simulink library "ddm"  (R2021b)
settings: Solver=VariableStepAuto  StartTime=0.0  StopTime=10.0  RelTol=1e-3
undefined symbols (not defined in the file or in its folder): ADDM_FrTMTqDev_X_Nm, ADDM_RrTMTqDev_X_Nm, ENUM_ADASACCSTA_ERROR, ENUM_ADASACCSTA_OFF, ENUM_ADASACCSTA_STANDBY, ENUM_ALLOWMOV_ALLOWREADY, ENUM_APS, ENUM_BRKSTA_ERROR, ENUM_BRKSTA_OFF, ENUM_BRKSTA_ON, ENUM_BRKSW_INVALID, ENUM_BRKSW_OFF, ENUM_BRKSW_ON, ENUM_CHGPREACTERRSTA_OBCPRE, ENUM_DCDCFAULTSTA_ANYFAULTLV1, ENUM_DCDCFAULTSTA_ANYFAULTLV2, ENUM_DRIVETRAIN_AWD, ENUM_DRIVETRAIN_FWD, ENUM_DRIVETRAIN_RWD, ENUM_EDUDRTSTA_NORMAL, ENUM_EPBSTA_APPLIED, ENUM_EPBSTA_RELEASED, ENUM_ESCAPSSta_APSUNAVAILABLE, ENUM_GEARACTUALPOSN_INVALID, ENUM_GEARACTUALPOSN_P, ENUM_HVBATTREADYPRE_READY, ENUM_MCUWARN_LV0, ENUM_MCUWARN_LV1, ENUM_MCUWARN_LV2, ENUM_MCUWARN_LV3, ENUM_MCUWARN_NOERROR, ENUM_OBCFAULTSTA_ANYFAULT, ENUM_PAS_R2F2, ENUM_PDFAULT_BATTPDFAIL, ENUM_PDFAULT_DCDCDISABLE, ENUM_PDFAULT_MCUDISABLE, ENUM_PDFAULT_MCUDISCHRG, ENUM_POWERSTA_OFF, ENUM_POWERSTA_ON, ENUM_POWERSTA_READY, ENUM_POWERSTA_STANDBY, ENUM_PRESSINDI_LOW, ENUM_PUFAULT_BATTUPFAIL, ENUM_PUFAULT_DCDCENABLEFAIL, ENUM_PUFAULT_PRECHRGCHKFAIL, ENUM_PUFAULT_SAFETYCHKFAIL, ENUM_PUSTATE_COMPLETED, ENUM_PWRSTASW_OFF, ENUM_PWRSTASW_OFFA, ENUM_PWRSTASW_OFFCHVCHRG, ENUM_PWRSTASW_OFFCLVCHRG, ENUM_PWRSTASW_ON, ENUM_PWRSTASW_ONHVCHRG, ENUM_PWRSTASW_READY, ENUM_PWRSTASW_STANDBY, ENUM_RAPSErrWarnSta_NORMAL, ENUM_RAPSErrWarnSta_RAPSERRLV1, ENUM_SHIFTCOMMAND_P, ENUM_SHIFTERERRSTA_PBUTTONFAILURE, ENUM_VEHMALFUNLV_2ND ... (+463)
libraries: hcu_lib x529, $bdroot x5, simulink x4
(part 18 of 25)

== system ddm/DDM/DDM/PMM/Comm err/VCU lost communication with ABM1 ==
  note: Test Detection Criteria
  note: Test Pass Criteria
  note: Release Condition After Decision
  note: Diagnostics and Fault Handling
  task_time_s : Inport
  VPMM_PowerSta_enum : Inport  Port=2
  VPMM_PwrStaSW_enum : Inport  Port=3
  VDDM_C1ABM1LCChk_flg : Inport  Port=4
  No_CAN1_BUS_OFF : Inport  Port=5
  DTC_clear_request : Inport  Port=6
  Constant1 : Constant  Value=ENUM_PWRSTASW_OFF
  Constant10 : Constant  Value=ENUM_POWERSTA_STANDBY
  Constant11 : Constant  Value=ZERO_INT
  Constant12 : Constant  Value=KDDM_C1ABM1LCDTC_cnt
  Constant13 : Constant  Value=FALSE
  Constant14 : Constant  Value=KDDM_C1ABM1LCDetTO_s
  Constant17 : Constant  Value=KDDM_C1ABM1LCDTC_cnt
  Constant29 : Constant  Value=FALSE
  Constant30 : Constant  Value=KDDM_CommErrDiagnosisOffSW_flg
  Constant31 : Constant  Value=ENUM_POWERSTA_OFF
  Constant6 : Constant  Value=KDDM_C1ABM1LCPassTO_s
  Constant7 : Constant  Value=TRUE
  Constant8 : Constant  Value=KDDM_C1ABM1LCPassTO_s
  Constant9 : Constant  Value=ENUM_PWRSTASW_OFF
  DTC_Couter1 : hcu_lib/Basic_Blocks/DTC_Couter
  DTC_Info : hcu_lib/Basic_Blocks/DTC_Info
  Equal1 : RelationalOperator  Operator=~=  OutDataTypeStr=boolean  RndMeth=Simplest
  Equal5 : RelationalOperator  Operator=~=  OutDataTypeStr=boolean  RndMeth=Simplest
  Equal6 : RelationalOperator  OutDataTypeStr=boolean  RndMeth=Simplest
  Equal7 : RelationalOperator  Operator===  OutDataTypeStr=boolean  RndMeth=Simplest
  Equal8 : RelationalOperator  Operator===  OutDataTypeStr=boolean  RndMeth=Simplest
  Logical Operator1 : Logic  Operator=NOT  AllPortsSameDT=off  OutDataTypeStr=boolean
  Logical Operator10 : Logic  AllPortsSameDT=off  OutDataTypeStr=boolean
  Logical Operator14 : Logic  Operator=OR  Inputs=4  AllPortsSameDT=off  OutDataTypeStr=boolean
  Logical Operator16 : Logic  AllPortsSameDT=off  OutDataTypeStr=boolean
  Logical Operator20 : Logic  Operator=NOT  AllPortsSameDT=off  OutDataTypeStr=boolean
  Logical Operator3 : Logic  Operator=NOT  AllPortsSameDT=off  OutDataTypeStr=boolean
  Logical Operator9 : Logic  AllPortsSameDT=off  OutDataTypeStr=boolean
  Relational Operator1 : RelationalOperator  Operator=>  OutDataTypeStr=boolean  RndMeth=Simplest
  Switch2 : Switch  Criteria=u2 ~= 0
  Switch8 : Switch  Criteria=u2 ~= 0
  Switch9 : Switch  Criteria=u2 ~= 0
  Terminator : Terminator
  Test Detection Criteria1 : hcu_lib/Basic_Blocks/Test Detection Criteria
  Timer2 : hcu_lib/Basic_Blocks/Timer
  Unit Delay1 : UnitDelay  SampleTime=-1  HasFrameUpgradeWarning=on
  VDDM_C1ABM1LCDTC_raw32 : Outport
  VDDM_C1ABM1LCCFS_flg : Outport  Port=2
  LC_EDriveSysErr_VCUErr_flg : Outport  Port=3
  wires:
  [DTC_clear_request] -> DTC_Info/4
  [VDDM_C1ABM1LCPass_flg] -> DTC_Info/2
  [VDDM_C1ABM1LCDet_flg] -> DTC_Info/1
  [VDDM_C1ABM1LCCFS_flg] -> DTC_Info/3
  DTC_Info/1 -> VDDM_C1ABM1LCDTC_raw32/1  "VDDM_C1ABM1LCDTC_raw32"
  [VDDM_C1ABM1LCCFS_flg] -> LC_EDriveSysErr_VCUErr_flg/1, VDDM_C1ABM1LCCFS_flg/1
  No_CAN1_BUS_OFF/1 -> [No_CAN1_BUS_OFF]
  DTC_clear_request/1 -> [DTC_clear_request]
  task_time_s/1 -> [task_time_s]
  VDDM_C1ABM1LCChk_flg/1 -> [VDDM_C1ABM1LCChk_flg]
  VPMM_PwrStaSW_enum/1 -> [VPMM_PwrStaSW_enum]
  VPMM_PowerSta_enum/1 -> [VPMM_PowerSta_enum]
  [VDDM_C1ABM1LCCFSRls_flg] -> Switch9/2
  [VDDM_C1ABM1LCChk_flg] -> Logical Operator1/1
  [VDDM_C1ABM1LCChk_flg] -> Logical Operator3/1
  [VDDM_C1ABM1LCCFSRls_flg] -> DTC_Couter1/2
  [task_time_s] -> Test Detection Criteria1/2
  Logical Operator20/1 -> Timer2/1
  [VPMM_PwrStaSW_enum] -> Equal5/1
  Logical Operator10/1 -> Switch8/2
  [No_CAN1_BUS_OFF] -> Logical Operator10/1
  Constant1/1 -> Equal5/2
  Relational Operator1/1 -> Terminator/1  "VDDM_C1ABM1LCDFS_flg"
  Constant6/1 -> Timer2/4
  Constant14/1 -> Test Detection Criteria1/4
  Constant10/1 -> Equal8/2
  Logical Operator16/1 -> Logical Operator14/1
  Equal7/1 -> Logical Operator16/1
  Constant12/1 -> Test Detection Criteria1/3
  [task_time_s] -> Timer2/3
  Equal5/1 -> Logical Operator10/2
  Equal6/1 -> [VDDM_C1ABM1LCPass_flg]  "VDDM_C1ABM1LCPass_flg"
  Constant17/1 -> DTC_Couter1/3
  Equal8/1 -> Logical Operator16/2
  Constant11/1 -> Relational Operator1/2
  [No_CAN1_BUS_OFF] -> Logical Operator9/1
  [VDDM_C1ABM1LCPass_flg] -> Logical Operator14/3
  Switch9/1 -> Test Detection Criteria1/1
  [VDDM_C1ABM1LCDet_flg] -> DTC_Couter1/1
  Constant31/1 -> Equal7/2
  DTC_Couter1/2 -> Relational Operator1/1  "VDDM_C1ABM1LCDTC_cnt"
  DTC_Couter1/1 -> [VDDM_C1ABM1LCCFS_flg]  "VDDM_C1ABM1LCCFS_flg"
  Unit Delay1/1 -> Equal7/1
  Constant13/1 -> Switch2/3
  [DTC_clear_request] -> Logical Operator14/2
  Constant9/1 -> Equal1/2
  Constant8/1 -> Equal6/2
  Constant7/1 -> Switch8/3
  [VPMM_PowerSta_enum] -> Equal8/1
  Timer2/1 -> Equal6/1
  [VPMM_PwrStaSW_enum] -> Equal1/1
  Logical Operator14/1 -> [VDDM_C1ABM1LCCFSRls_flg]  "VDDM_C1ABM1LCCFSRls_flg"
  Constant30/1 -> Logical Operator14/4
  Switch8/1 -> Timer2/2, Logical Operator20/1
  Logical Operator9/1 -> Switch2/2
  Test Detection Criteria1/1 -> [VDDM_C1ABM1LCDet_flg]  "VDDM_C1ABM1LCDet_flg"
  Constant29/1 -> Switch9/1
  Equal1/1 -> Logical Operator9/2
  [VPMM_PowerSta_enum] -> Unit Delay1/1
  Switch2/1 -> Switch9/3
  Logical Operator3/1 -> Switch2/1
  Logical Operator1/1 -> Switch8/1

== system ddm/DDM/DDM/PMM/Comm err/VCU lost communication with BMS1 ==
  note: Test Pass Criteria
  note: Test Detection Criteria
  note: Diagnostics and Fault Handling
  note: Release Condition After Decision
  task_time_s : Inport
  VPMM_PowerSta_enum : Inport  Port=2
  VPMM_PwrStaSW_enum : Inport  Port=3
  VDDM_C3BMS1LCChk_flg : Inport  Port=4
  No_CAN3_BUS_OFF : Inport  Port=5
  DTC_clear_request : Inport  Port=6
  Constant1 : Constant  Value=ENUM_PWRSTASW_OFF
  Constant10 : Constant  Value=ENUM_POWERSTA_STANDBY
  Constant11 : Constant  Value=ZERO_INT
  Constant12 : Constant  Value=KDDM_C3BMS1LCPassTO_s
  Constant13 : Constant  Value=FALSE
  Constant14 : Constant  Value=KDDM_C3BMS1LCDTC_cnt
  Constant17 : Constant  Value=KDDM_C3BMS1LCDetTO_s
  Constant29 : Constant  Value=FALSE
  Constant30 : Constant  Value=KDDM_CommErrDiagnosisOffSW_flg
  Constant31 : Constant  Value=ENUM_POWERSTA_OFF
  Constant6 : Constant  Value=KDDM_C3BMS1LCDTC_cnt
  Constant7 : Constant  Value=TRUE
  Constant8 : Constant  Value=KDDM_C3BMS1LCPassTO_s
  Constant9 : Constant  Value=ENUM_PWRSTASW_OFF
  DTC_Couter1 : hcu_lib/Basic_Blocks/DTC_Couter
  DTC_Info : hcu_lib/Basic_Blocks/DTC_Info
  Delay1 : Delay  DelayLength=1
  Equal1 : RelationalOperator  Operator=~=  OutDataTypeStr=boolean  RndMeth=Simplest
  Equal5 : RelationalOperator  Operator=~=  OutDataTypeStr=boolean  RndMeth=Simplest
  Equal6 : RelationalOperator  OutDataTypeStr=boolean  RndMeth=Simplest
  Equal7 : RelationalOperator  Operator===  OutDataTypeStr=boolean  RndMeth=Simplest
  Equal8 : RelationalOperator  Operator===  OutDataTypeStr=boolean  RndMeth=Simplest
  Logical Operator : Logic  Operator=NOT  AllPortsSameDT=off  OutDataTypeStr=boolean
  Logical Operator14 : Logic  Operator=OR  Inputs=4  AllPortsSameDT=off  OutDataTypeStr=boolean
  Logical Operator{7,9,16,22} (4 alike) : Logic  AllPortsSameDT=off  OutDataTypeStr=boolean
  Logical Operator2 : Logic  Operator=NOT  AllPortsSameDT=off  OutDataTypeStr=boolean
  Logical Operator20 : Logic  Operator=NOT  AllPortsSameDT=off  OutDataTypeStr=boolean
  NOT1 : Logic  Operator=NOT  AllPortsSameDT=off  OutDataTypeStr=boolean
  Relational Operator1 : RelationalOperator  Operator=>  OutDataTypeStr=boolean  RndMeth=Simplest
  Switch2 : Switch  Criteria=u2 ~= 0
  Switch8 : Switch  Criteria=u2 ~= 0
  Switch9 : Switch  Criteria=u2 ~= 0
  Terminator : Terminator
  Test Detection Criteria1 : hcu_lib/Basic_Blocks/Test Detection Criteria
  Timer2 : hcu_lib/Basic_Blocks/Timer
  Unit Delay1 : UnitDelay  SampleTime=-1  HasFrameUpgradeWarning=on
  VDDM_C3BMS1LCDTC_raw32 : Outport
  VDDM_C3BMS1LCCFS_flg : Outport  Port=2
  wires:
  [VDDM_C3BMS1LCCFS_flg] -> Delay1/1
  Logical Operator20/1 -> Timer2/1
  Logical Operator14/1 -> [VDDM_C3BMS1LCCFSRls_flg]  "VDDM_C3BMS1LCCFSRls_flg"
  [task_time_s] -> Test Detection Criteria1/2
  Timer2/1 -> Equal6/1
  Test Detection Criteria1/1 -> [VDDM_C3BMS1LCDet_flg]  "VDDM_C3BMS1LCDet_flg"
  Equal1/1 -> Logical Operator7/2
  Constant9/1 -> Equal1/2
  Constant10/1 -> Equal8/2
  Constant8/1 -> Timer2/4
  Relational Operator1/1 -> Terminator/1  "VDDM_C3BMS1LCDFS_flg"
  Constant1/1 -> Equal5/2
  [No_CAN3_BUS_OFF] -> Logical Operator7/1
  Logical Operator16/1 -> Logical Operator14/1
  [VPMM_PwrStaSW_enum] -> Equal1/1
  DTC_Couter1/1 -> [VDDM_C3BMS1LCCFS_flg]  "VDDM_C3BMS1LCCFS_flg"
  [VPMM_PwrStaSW_enum] -> Equal5/1
  Equal5/1 -> Logical Operator9/2
  [No_CAN3_BUS_OFF] -> Logical Operator9/1
  Logical Operator7/1 -> Switch2/2
  [VDDM_C3BMS1LCPass_flg] -> Logical Operator22/1
  Delay1/1 -> NOT1/1
  Constant12/1 -> Equal6/2
  Unit Delay1/1 -> Equal7/1
  [VDDM_C3BMS1LCChk_flg] -> Logical Operator2/1
  Switch2/1 -> Switch9/3
  [task_time_s] -> Timer2/3
  [VDDM_C3BMS1LCDet_flg] -> DTC_Couter1/1
  Logical Operator9/1 -> Switch8/2
  [VDDM_C3BMS1LCChk_flg] -> Logical Operator/1
  [VDDM_C3BMS1LCCFSRls_flg] -> Switch9/2
  Equal6/1 -> [VDDM_C3BMS1LCPass_flg]  "VDDM_C3BMS1LCPass_flg"
  Constant6/1 -> DTC_Couter1/3
  Constant7/1 -> Switch8/3
  Logical Operator22/1 -> Logical Operator14/3
  Switch9/1 -> Test Detection Criteria1/1
  Constant30/1 -> Logical Operator14/4
  Equal8/1 -> Logical Operator16/2
  Constant29/1 -> Switch9/1
  NOT1/1 -> Logical Operator22/2
  [VPMM_PowerSta_enum] -> Equal8/1
  Constant13/1 -> Switch2/3
  Constant11/1 -> Relational Operator1/2
  DTC_Couter1/2 -> Relational Operator1/1  "VDDM_C3BMS1LCDTC_cnt"
  [DTC_clear_request] -> Logical Operator14/2
  Switch8/1 -> Logical Operator20/1, Timer2/2
  Constant31/1 -> Equal7/2
  [VPMM_PowerSta_enum] -> Unit Delay1/1
  Equal7/1 -> Logical Operator16/1
  [VDDM_C3BMS1LCCFSRls_flg] -> DTC_Couter1/2
  Constant14/1 -> Test Detection Criteria1/3
  Constant17/1 -> Test Detection Criteria1/4
  [VDDM_C3BMS1LCCFS_flg] -> DTC_Info/3, VDDM_C3BMS1LCCFS_flg/1
  task_time_s/1 -> [task_time_s]
  VDDM_C3BMS1LCChk_flg/1 -> [VDDM_C3BMS1LCChk_flg]
  VPMM_PwrStaSW_enum/1 -> [VPMM_PwrStaSW_enum]
  VPMM_PowerSta_enum/1 -> [VPMM_PowerSta_enum]
  No_CAN3_BUS_OFF/1 -> [No_CAN3_BUS_OFF]
  DTC_clear_request/1 -> [DTC_clear_request]
  DTC_Info/1 -> VDDM_C3BMS1LCDTC_raw32/1  "VDDM_C3BMS1LCDTC_raw32"
  [VDDM_C3BMS1LCDet_flg] -> DTC_Info/1
  [VDDM_C3BMS1LCPass_flg] -> DTC_Info/2
  [DTC_clear_request] -> DTC_Info/4
  Logical Operator/1 -> Switch2/1
  Logical Operator2/1 -> Switch8/1

== system ddm/DDM/DDM/PMM/Comm err/VCU lost communication with BMS6 ==
  note: Test Detection Criteria
  note: Release Condition After Decision
  note: Diagnostics and Fault Handling
  note: Test Pass Criteria
  task_time_s : Inport
  VPMM_PowerSta_enum : Inport  Port=2
  VPMM_PwrStaSW_enum : Inport  Port=3
  VDDM_C3BMS6LCChk_flg : Inport  Port=4
  No_CAN3_BUS_OFF : Inport  Port=5
  DTC_clear_request : Inport  Port=6
  Constant1 : Constant  Value=ENUM_PWRSTASW_OFF
  Constant10 : Constant  Value=ENUM_POWERSTA_STANDBY
  Constant11 : Constant  Value=ZERO_INT
  Constant12 : Constant  Value=KDDM_C3BMS6LCPassTO_s
  Constant13 : Constant  Value=FALSE
  Constant14 : Constant  Value=KDDM_C3BMS6LCDTC_cnt
  Constant17 : Constant  Value=KDDM_C3BMS6LCDetTO_s
  Constant27 : Constant  Value=KDDM_C3BMS6LCDTC_cnt
  Constant30 : Constant  Value=KDDM_CommErrDiagnosisOffSW_flg
  Constant31 : Constant  Value=ENUM_POWERSTA_OFF
  Constant6 : Constant  Value=TRUE
  Constant7 : Constant  Value=KDDM_C3BMS6LCPassTO_s
  Constant8 : Constant  Value=ENUM_PWRSTASW_OFF
  Constant9 : Constant  Value=FALSE
  DTC_Couter1 : hcu_lib/Basic_Blocks/DTC_Couter
  DTC_Info : hcu_lib/Basic_Blocks/DTC_Info
  Delay1 : Delay  DelayLength=1
  Equal1 : RelationalOperator  Operator=~=  OutDataTypeStr=boolean  RndMeth=Simplest
  Equal5 : RelationalOperator  Operator=~=  OutDataTypeStr=boolean  RndMeth=Simplest
  Equal6 : RelationalOperator  OutDataTypeStr=boolean  RndMeth=Simplest
  Equal7 : RelationalOperator  Operator===  OutDataTypeStr=boolean  RndMeth=Simplest
  Equal8 : RelationalOperator  Operator===  OutDataTypeStr=boolean  RndMeth=Simplest
  Logical Operator : Logic  Operator=NOT  AllPortsSameDT=off  OutDataTypeStr=boolean
  Logical Operator14 : Logic  Operator=OR  Inputs=4  AllPortsSameDT=off  OutDataTypeStr=boolean
  Logical Operator{7,9,16,22} (4 alike) : Logic  AllPortsSameDT=off  OutDataTypeStr=boolean
  Logical Operator2 : Logic  Operator=NOT  AllPortsSameDT=off  OutDataTypeStr=boolean
  Logical Operator20 : Logic  Operator=NOT  AllPortsSameDT=off  OutDataTypeStr=boolean
  NOT1 : Logic  Operator=NOT  AllPortsSameDT=off  OutDataTypeStr=boolean
  Relational Operator1 : RelationalOperator  Operator=>  OutDataTypeStr=boolean  RndMeth=Simplest
  Switch2 : Switch  Criteria=u2 ~= 0
  Switch8 : Switch  Criteria=u2 ~= 0
  Switch9 : Switch  Criteria=u2 ~= 0
  Terminator : Terminator
  Test Detection Criteria1 : hcu_lib/Basic_Blocks/Test Detection Criteria
  Timer2 : hcu_lib/Basic_Blocks/Timer
  Unit Delay1 : UnitDelay  SampleTime=-1  HasFrameUpgradeWarning=on
  VDDM_C3BMS6LCDTC_raw32 : Outport
  VDDM_C3BMS6LCCFS_flg : Outport  Port=2
  wires:
  Equal5/1 -> Logical Operator9/2
  Constant1/1 -> Equal5/2
  [No_CAN3_BUS_OFF] -> Logical Operator9/1
  [VPMM_PwrStaSW_enum] -> Equal5/1
  Equal1/1 -> Logical Operator7/2
  [VPMM_PwrStaSW_enum] -> Equal1/1
  Constant8/1 -> Equal1/2
  [No_CAN3_BUS_OFF] -> Logical Operator7/1
  [task_time_s] -> Timer2/3
  Timer2/1 -> Equal6/1
  [VDDM_C3BMS6LCChk_flg] -> Logical Operator/1
  Logical Operator20/1 -> Timer2/1
  Logical Operator16/1 -> Logical Operator14/1
  Relational Operator1/1 -> Terminator/1  "VDDM_C3BMS6LCDFS_flg"
  Constant27/1 -> DTC_Couter1/3
  Test Detection Criteria1/1 -> [VDDM_C3BMS6LCDet_flg]  "VDDM_C3BMS6LCDet_flg"
  [VDDM_C3BMS6LCChk_flg] -> Logical Operator2/1
  [VDDM_C3BMS6LCCFS_flg] -> Delay1/1
  Equal7/1 -> Logical Operator16/1
  Equal6/1 -> [VDDM_C3BMS6LCPass_flg]  "VDDM_C3BMS6LCPass_flg"
  [VPMM_PowerSta_enum] -> Unit Delay1/1
  [VDDM_C3BMS6LCDet_flg] -> DTC_Couter1/1
  DTC_Couter1/1 -> [VDDM_C3BMS6LCCFS_flg]  "VDDM_C3BMS6LCCFS_flg"
  Constant31/1 -> Equal7/2
  [VDDM_C3BMS6LCPass_flg] -> Logical Operator22/1
  Constant17/1 -> Test Detection Criteria1/4
  Constant14/1 -> Test Detection Criteria1/3
  Unit Delay1/1 -> Equal7/1
  Switch8/1 -> Logical Operator20/1, Timer2/2
  [DTC_clear_request] -> Logical Operator14/2
  Constant7/1 -> Timer2/4
  [VDDM_C3BMS6LCCFSRls_flg] -> DTC_Couter1/2
  Delay1/1 -> NOT1/1
  DTC_Couter1/2 -> Relational Operator1/1  "VDDM_C3BMS6LCDTC_cnt"
  Constant11/1 -> Relational Operator1/2
  Constant13/1 -> Switch2/3
  Logical Operator9/1 -> Switch8/2
  Constant10/1 -> Equal8/2
  Constant9/1 -> Switch9/1
  Switch2/1 -> Switch9/3
  [task_time_s] -> Test Detection Criteria1/2
  [VPMM_PowerSta_enum] -> Equal8/1
  Equal8/1 -> Logical Operator16/2
  Logical Operator7/1 -> Switch2/2
  NOT1/1 -> Logical Operator22/2
  Logical Operator22/1 -> Logical Operator14/3
  Constant6/1 -> Switch8/3
  Constant30/1 -> Logical Operator14/4
  Switch9/1 -> Test Detection Criteria1/1
  Logical Operator14/1 -> [VDDM_C3BMS6LCCFSRls_flg]  "VDDM_C3BMS6LCCFSRls_flg"
  Constant12/1 -> Equal6/2
  [VDDM_C3BMS6LCCFSRls_flg] -> Switch9/2
  VPMM_PowerSta_enum/1 -> [VPMM_PowerSta_enum]
  VPMM_PwrStaSW_enum/1 -> [VPMM_PwrStaSW_enum]
  VDDM_C3BMS6LCChk_flg/1 -> [VDDM_C3BMS6LCChk_flg]
  task_time_s/1 -> [task_time_s]
  [VDDM_C3BMS6LCCFS_flg] -> DTC_Info/3, VDDM_C3BMS6LCCFS_flg/1
  DTC_clear_request/1 -> [DTC_clear_request]
  No_CAN3_BUS_OFF/1 -> [No_CAN3_BUS_OFF]
  [VDDM_C3BMS6LCPass_flg] -> DTC_Info/2
  DTC_Info/1 -> VDDM_C3BMS6LCDTC_raw32/1  "VDDM_C3BMS6LCDTC_raw32"
  [VDDM_C3BMS6LCDet_flg] -> DTC_Info/1
  [DTC_clear_request] -> DTC_Info/4
  Logical Operator/1 -> Switch2/1
  Logical Operator2/1 -> Switch8/1

== system ddm/DDM/DDM/PMM/Comm err/VCU lost communication with CCU1 ==
  note: Diagnostics and Fault Handling
  note: Test Pass Criteria
  note: Test Detection Criteria
  note: Release Condition After Decision
  task_time_s : Inport
  VPMM_PowerSta_enum : Inport  Port=2
  VPMM_PwrStaSW_enum : Inport  Port=3
  VDDM_C3CCU1LCChk_flg : Inport  Port=4
  No_CAN3_BUS_OFF : Inport  Port=5
  DTC_clear_request : Inport  Port=6
  Constant1 : Constant  Value=ENUM_PWRSTASW_OFF
  Constant10 : Constant  Value=ENUM_POWERSTA_STANDBY
  Constant11 : Constant  Value=ZERO_INT
  Constant12 : Constant  Value=KDDM_C3CCU1LCPassTO_s
  Constant13 : Constant  Value=FALSE
  Constant14 : Constant  Value=KDDM_C3CCU1LCDTC_cnt
  Constant17 : Constant  Value=KDDM_C3CCU1LCDetTO_s
  Constant29 : Constant  Value=FALSE
  Constant30 : Constant  Value=KDDM_CommErrDiagnosisOffSW_flg
  Constant31 : Constant  Value=ENUM_POWERSTA_OFF
  Constant32 : Constant  Value=KDDM_C3CCU1LCDTC_cnt
  Constant7 : Constant  Value=TRUE
  Constant8 : Constant  Value=KDDM_C3CCU1LCPassTO_s
  Constant9 : Constant  Value=ENUM_PWRSTASW_OFF
  DTC_Couter1 : hcu_lib/Basic_Blocks/DTC_Couter
  DTC_Info : hcu_lib/Basic_Blocks/DTC_Info
  Delay1 : Delay  DelayLength=1
  Equal1 : RelationalOperator  Operator=~=  OutDataTypeStr=boolean  RndMeth=Simplest
  Equal5 : RelationalOperator  Operator=~=  OutDataTypeStr=boolean  RndMeth=Simplest
  Equal6 : RelationalOperator  OutDataTypeStr=boolean  RndMeth=Simplest
  Equal7 : RelationalOperator  Operator===  OutDataTypeStr=boolean  RndMeth=Simplest
  Equal8 : RelationalOperator  Operator===  OutDataTypeStr=boolean  RndMeth=Simplest
  Logical Operator1 : Logic  Operator=NOT  AllPortsSameDT=off  OutDataTypeStr=boolean
  Logical Operator14 : Logic  Operator=OR  Inputs=4  AllPortsSameDT=off  OutDataTypeStr=boolean
  Logical Operator{7,9,16,22} (4 alike) : Logic  AllPortsSameDT=off  OutDataTypeStr=boolean
  Logical Operator2 : Logic  Operator=NOT  AllPortsSameDT=off  OutDataTypeStr=boolean
  Logical Operator20 : Logic  Operator=NOT  AllPortsSameDT=off  OutDataTypeStr=boolean
  NOT1 : Logic  Operator=NOT  AllPortsSameDT=off  OutDataTypeStr=boolean
  Relational Operator1 : RelationalOperator  Operator=>  OutDataTypeStr=boolean  RndMeth=Simplest
  Switch2 : Switch  Criteria=u2 ~= 0
  Switch8 : Switch  Criteria=u2 ~= 0
  Switch9 : Switch  Criteria=u2 ~= 0
  Terminator : Terminator
  Test Detection Criteria1 : hcu_lib/Basic_Blocks/Test Detection Criteria
  Timer2 : hcu_lib/Basic_Blocks/Timer
  Unit Delay1 : UnitDelay  SampleTime=-1  HasFrameUpgradeWarning=on
  VDDM_C3CCU1LCDTC_raw32 : Outport
  VDDM_C3CCU1LCCFS_flg : Outport  Port=2
  wires:
  [DTC_clear_request] -> DTC_Info/4
  [VDDM_C3CCU1LCDet_flg] -> DTC_Info/1
  [VDDM_C3CCU1LCCFS_flg] -> VDDM_C3CCU1LCCFS_flg/1, DTC_Info/3
  [VDDM_C3CCU1LCPass_flg] -> DTC_Info/2
  DTC_Info/1 -> VDDM_C3CCU1LCDTC_raw32/1  "VDDM_C3CCU1LCDTC_raw32"
  No_CAN3_BUS_OFF/1 -> [No_CAN3_BUS_OFF]
  DTC_clear_request/1 -> [DTC_clear_request]
  task_time_s/1 -> [task_time_s]
  VDDM_C3CCU1LCChk_flg/1 -> [VDDM_C3CCU1LCChk_flg]
  VPMM_PwrStaSW_enum/1 -> [VPMM_PwrStaSW_enum]
  VPMM_PowerSta_enum/1 -> [VPMM_PowerSta_enum]
  Constant8/1 -> Timer2/4
  Relational Operator1/1 -> Terminator/1  "VDDM_C3CCU1LCDFS_flg"
  [No_CAN3_BUS_OFF] -> Logical Operator9/1
  Test Detection Criteria1/1 -> [VDDM_C3CCU1LCDet_flg]  "VDDM_C3CCU1LCDet_flg"
  Logical Operator16/1 -> Logical Operator14/1
  Constant10/1 -> Equal8/2
  [VPMM_PwrStaSW_enum] -> Equal1/1
  [task_time_s] -> Timer2/3
  Constant12/1 -> Equal6/2
  Switch2/1 -> Switch9/3
  Equal5/1 -> Logical Operator9/2
  Logical Operator7/1 -> Switch2/2
  Delay1/1 -> NOT1/1
  Constant32/1 -> DTC_Couter1/3
  Constant7/1 -> Switch8/3
  Constant30/1 -> Logical Operator14/4
  Constant29/1 -> Switch9/1
  [VPMM_PowerSta_enum] -> Equal8/1
  Constant13/1 -> Switch2/3
  Switch9/1 -> Test Detection Criteria1/1
  DTC_Couter1/1 -> [VDDM_C3CCU1LCCFS_flg]  "VDDM_C3CCU1LCCFS_flg"
  Logical Operator22/1 -> Logical Operator14/3
  Equal8/1 -> Logical Operator16/2
  Constant11/1 -> Relational Operator1/2
  NOT1/1 -> Logical Operator22/2
  [DTC_clear_request] -> Logical Operator14/2
  Unit Delay1/1 -> Equal7/1
  DTC_Couter1/2 -> Relational Operator1/1  "VDDM_C3CCU1LCDTC_cnt"
  Timer2/1 -> Equal6/1
  Constant31/1 -> Equal7/2
  [VPMM_PowerSta_enum] -> Unit Delay1/1
  Switch8/1 -> Timer2/2, Logical Operator20/1
  Constant17/1 -> Test Detection Criteria1/4
  Equal1/1 -> Logical Operator7/2
  Equal7/1 -> Logical Operator16/1
  [VDDM_C3CCU1LCChk_flg] -> Logical Operator2/1
  [VPMM_PwrStaSW_enum] -> Equal5/1
  Logical Operator20/1 -> Timer2/1
  Constant14/1 -> Test Detection Criteria1/3
  [VDDM_C3CCU1LCPass_flg] -> Logical Operator22/1
  Logical Operator9/1 -> Switch8/2
  Logical Operator14/1 -> [VDDM_C3CCU1LCCFSRls_flg]  "VDDM_C3CCU1LCCFSRls_flg"
  Constant9/1 -> Equal1/2
  [task_time_s] -> Test Detection Criteria1/2
  [No_CAN3_BUS_OFF] -> Logical Operator7/1
  [VDDM_C3CCU1LCChk_flg] -> Logical Operator1/1
  [VDDM_C3CCU1LCCFSRls_flg] -> DTC_Couter1/2
  Constant1/1 -> Equal5/2
  [VDDM_C3CCU1LCCFS_flg] -> Delay1/1
  [VDDM_C3CCU1LCDet_flg] -> DTC_Couter1/1
  [VDDM_C3CCU1LCCFSRls_flg] -> Switch9/2
  Equal6/1 -> [VDDM_C3CCU1LCPass_flg]  "VDDM_C3CCU1LCPass_flg"
  Logical Operator2/1 -> Switch2/1
  Logical Operator1/1 -> Switch8/1

== system ddm/DDM/DDM/PMM/Comm err/VCU lost communication with CCU2 ==
  note: Test Detection Criteria
  note: Test Pass Criteria
  note: Diagnostics and Fault Handling
  note: Release Condition After Decision
  task_time_s : Inport
  VPMM_PowerSta_enum : Inport  Port=2
  VPMM_PwrStaSW_enum : Inport  Port=3
  VDDM_C3CCU2LCChk_flg : Inport  Port=4
  No_CAN3_BUS_OFF : Inport  Port=5
  DTC_clear_request : Inport  Port=6
  Constant1 : Constant  Value=ENUM_PWRSTASW_OFF
  Constant10 : Constant  Value=ENUM_POWERSTA_STANDBY
  Constant11 : Constant  Value=ZERO_INT
  Constant12 : Constant  Value=KDDM_C3CCU2LCPassTO_s
  Constant13 : Constant  Value=FALSE
  Constant14 : Constant  Value=KDDM_C3CCU2LCDTC_cnt
  Constant17 : Constant  Value=KDDM_C3CCU2LCDetTO_s
  Constant29 : Constant  Value=FALSE
  Constant30 : Constant  Value=KDDM_CommErrDiagnosisOffSW_flg
  Constant31 : Constant  Value=ENUM_POWERSTA_OFF
  Constant32 : Constant  Value=KDDM_C3CCU2LCDTC_cnt
  Constant7 : Constant  Value=TRUE
  Constant8 : Constant  Value=KDDM_C3CCU2LCPassTO_s
  Constant9 : Constant  Value=ENUM_PWRSTASW_OFF
  DTC_Couter1 : hcu_lib/Basic_Blocks/DTC_Couter
  DTC_Info : hcu_lib/Basic_Blocks/DTC_Info
  Delay1 : Delay  DelayLength=1
  Equal1 : RelationalOperator  Operator=~=  OutDataTypeStr=boolean  RndMeth=Simplest
  Equal5 : RelationalOperator  Operator=~=  OutDataTypeStr=boolean  RndMeth=Simplest
  Equal6 : RelationalOperator  OutDataTypeStr=boolean  RndMeth=Simplest
  Equal7 : RelationalOperator  Operator===  OutDataTypeStr=boolean  RndMeth=Simplest
  Equal8 : RelationalOperator  Operator===  OutDataTypeStr=boolean  RndMeth=Simplest
  Logical Operator1 : Logic  Operator=NOT  AllPortsSameDT=off  OutDataTypeStr=boolean
  Logical Operator14 : Logic  Operator=OR  Inputs=4  AllPortsSameDT=off  OutDataTypeStr=boolean
  Logical Operator{7,9,16,22} (4 alike) : Logic  AllPortsSameDT=off  OutDataTypeStr=boolean
  Logical Operator20 : Logic  Operator=NOT  AllPortsSameDT=off  OutDataTypeStr=boolean
  Logical Operator3 : Logic  Operator=NOT  AllPortsSameDT=off  OutDataTypeStr=boolean
  NOT1 : Logic  Operator=NOT  AllPortsSameDT=off  OutDataTypeStr=boolean
  Relational Operator1 : RelationalOperator  Operator=>  OutDataTypeStr=boolean  RndMeth=Simplest
  Switch2 : Switch  Criteria=u2 ~= 0
  Switch8 : Switch  Criteria=u2 ~= 0
  Switch9 : Switch  Criteria=u2 ~= 0
  Terminator : Terminator
  Test Detection Criteria1 : hcu_lib/Basic_Blocks/Test Detection Criteria
  Timer2 : hcu_lib/Basic_Blocks/Timer
  Unit Delay1 : UnitDelay  SampleTime=-1  HasFrameUpgradeWarning=on
  VDDM_C3CCU2LCDTC_raw32 : Outport
  VDDM_C3CCU2LCCFS_flg : Outport  Port=2
  wires:
  [DTC_clear_request] -> DTC_Info/4
  [VDDM_C3CCU2LCDet_flg] -> DTC_Info/1
  [VDDM_C3CCU2LCCFS_flg] -> VDDM_C3CCU2LCCFS_flg/1, DTC_Info/3
  [VDDM_C3CCU2LCPass_flg] -> DTC_Info/2
  DTC_Info/1 -> VDDM_C3CCU2LCDTC_raw32/1  "VDDM_C3CCU2LCDTC_raw32"
  DTC_clear_request/1 -> [DTC_clear_request]
  No_CAN3_BUS_OFF/1 -> [No_CAN3_BUS_OFF]
  VPMM_PowerSta_enum/1 -> [VPMM_PowerSta_enum]
  VPMM_PwrStaSW_enum/1 -> [VPMM_PwrStaSW_enum]
  VDDM_C3CCU2LCChk_flg/1 -> [VDDM_C3CCU2LCChk_flg]
  task_time_s/1 -> [task_time_s]
  Constant14/1 -> Test Detection Criteria1/3
  Constant17/1 -> Test Detection Criteria1/4
  Constant8/1 -> Timer2/4
  [VDDM_C3CCU2LCPass_flg] -> Logical Operator22/1
  Logical Operator16/1 -> Logical Operator14/1
  Constant10/1 -> Equal8/2
  [No_CAN3_BUS_OFF] -> Logical Operator9/1
  Relational Operator1/1 -> Terminator/1  "VDDM_C3CCU2LCDFS_flg"
  Constant1/1 -> Equal5/2
  [VPMM_PwrStaSW_enum] -> Equal1/1
  [No_CAN3_BUS_OFF] -> Logical Operator7/1
  [VDDM_C3CCU2LCDet_flg] -> DTC_Couter1/1
  [VDDM_C3CCU2LCChk_flg] -> Logical Operator3/1
  [task_time_s] -> Test Detection Criteria1/2
  Logical Operator20/1 -> Timer2/1
  [VPMM_PwrStaSW_enum] -> Equal5/1
  Logical Operator9/1 -> Switch8/2
  Equal7/1 -> Logical Operator16/1
  [VDDM_C3CCU2LCCFS_flg] -> Delay1/1
  Switch8/1 -> Timer2/2, Logical Operator20/1
  Equal1/1 -> Logical Operator7/2
  [VPMM_PowerSta_enum] -> Unit Delay1/1
  Timer2/1 -> Equal6/1
  Constant12/1 -> Equal6/2
  Constant31/1 -> Equal7/2
  NOT1/1 -> Logical Operator22/2
  Constant9/1 -> Equal1/2
  [DTC_clear_request] -> Logical Operator14/2
  Unit Delay1/1 -> Equal7/1
  DTC_Couter1/2 -> Relational Operator1/1  "VDDM_C3CCU2LCDTC_cnt"
  Constant11/1 -> Relational Operator1/2
  Test Detection Criteria1/1 -> [VDDM_C3CCU2LCDet_flg]  "VDDM_C3CCU2LCDet_flg"
  Logical Operator22/1 -> Logical Operator14/3
  Equal8/1 -> Logical Operator16/2
  Switch9/1 -> Test Detection Criteria1/1
  [VDDM_C3CCU2LCCFSRls_flg] -> DTC_Couter1/2
  Constant13/1 -> Switch2/3
  Equal6/1 -> [VDDM_C3CCU2LCPass_flg]  "VDDM_C3CCU2LCPass_flg"
  Constant30/1 -> Logical Operator14/4
  Constant32/1 -> DTC_Couter1/3
  Constant7/1 -> Switch8/3
  [VPMM_PowerSta_enum] -> Equal8/1
  DTC_Couter1/1 -> [VDDM_C3CCU2LCCFS_flg]  "VDDM_C3CCU2LCCFS_flg"
  Equal5/1 -> Logical Operator9/2
  Logical Operator7/1 -> Switch2/2
  Delay1/1 -> NOT1/1
  [task_time_s] -> Timer2/3
  [VDDM_C3CCU2LCChk_flg] -> Logical Operator1/1
  Logical Operator14/1 -> [VDDM_C3CCU2LCCFSRls_flg]  "VDDM_C3CCU2LCCFSRls_flg"
  Switch2/1 -> Switch9/3
  Constant29/1 -> Switch9/1
  [VDDM_C3CCU2LCCFSRls_flg] -> Switch9/2
  Logical Operator3/1 -> Switch2/1
  Logical Operator1/1 -> Switch8/1

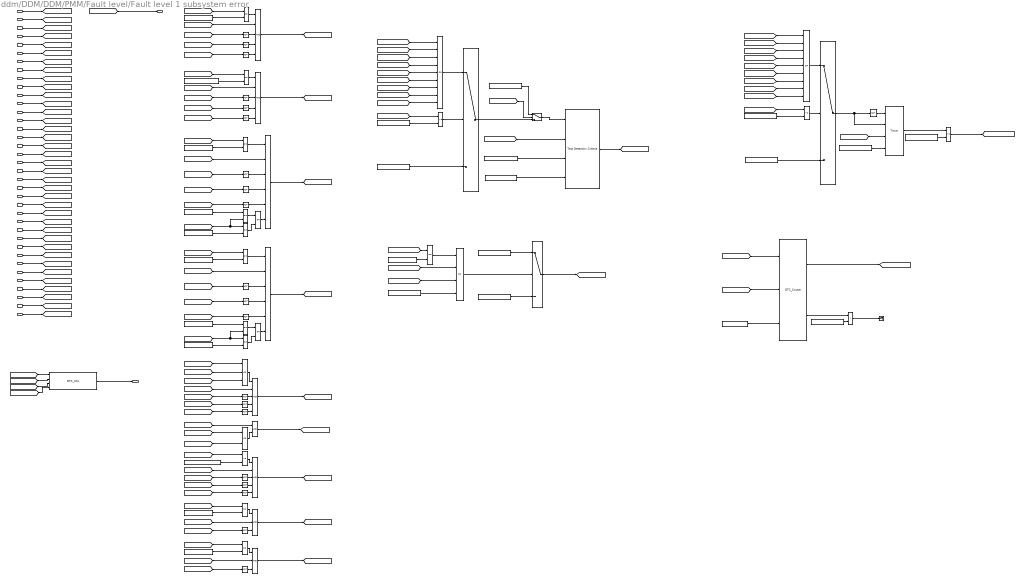
== system ddm/DDM/DDM/PMM/Fault level/Fault level 1 subsystem error ==
  note: VINP_MCUWarnFNidec_enum
  note: Release Condition After Failure Decision
  note: Diagnostics and Fault Handling
  note: Test Detection Criteria
  note: Test Pass Criteria
  task_time_s : Inport
  VPMM_PowerSta_enum : Inport  Port=2
  VPMM_PwrStaSW_enum : Inport  Port=3
  VDDM_C3BMS6LCCFS_flg : Inport  Port=4
  VDDM_C3CCU2LCCFS_flg : Inport  Port=5
  VDDM_MCUNF1NoComCFS_flg : Inport  Port=6
  VDDM_MCUNR1NoComCFS_flg : Inport  Port=7
  VINP_BMSWarn1_flg : Inport  Port=8
  VINP_BMSWarn2_flg : Inport  Port=9
  VINP_BMSWarn3_flg : Inport  Port=10
  VINP_DCDCFaultSta_enum : Inport  Port=11
  VINP_MCUWarnFNidec_enum : Inport  Port=12
  VINP_MCUWarnRNidec_enum : Inport  Port=13
  VINP_OBCFaultSta_enum : Inport  Port=14
  VPMM_DrivetrainSelect_enum : Inport  Port=15
  DTC_clear_request : Inport  Port=16
  No_CAN3_BUS_OFF : Inport  Port=17
  VDDM_C3CCU2RCCFS_flg : Inport  Port=18
  VDDM_C3CCU2CSCFS_flg : Inport  Port=19
  VDDM_MCUNR1RCErrCFS_flg : Inport  Port=20
  VDDM_MCUNR1CSErrCFS_flg : Inport  Port=21
  VDDM_MCUNF1RCErrCFS_flg : Inport  Port=22
  VDDM_MCUNF1CSErrCFS_flg : Inport  Port=23
  VDDM_C3BMS6RCCFS_flg : Inport  Port=24
  VDDM_C3BMS6CSCFS_flg : Inport  Port=25
  No_CAN1_BUS_OFF : Inport  Port=26
  VDDM_ESC1SigErr_flg : Inport  Port=27
  VDDM_ESC5SigErr_flg : Inport  Port=28
  VINP_ShifterFailsta_enum : Inport  Port=29
  VDDM_Shifter1NoComCFS_flg : Inport  Port=30
  VDDM_Shifter1RCErrCFS_flg : Inport  Port=31
  VDDM_Shifter1CSErrCFS_flg : Inport  Port=32
  VINP_ZoneDrMalfunLevel_enum : Inport  Port=33
  No_CAN4_BUS_OFF : Inport  Port=34
  VDDM_DrVCUNoComCFS_flg : Inport  Port=35
  ZoneFrMalfunLevel_enum : Inport  Port=36
  VDDM_FrVCUNoComCFS_flg : Inport  Port=37
  AND{,1..2,4} (4 alike) : Logic  Inputs=5  AllPortsSameDT=off  OutDataTypeStr=boolean
  AND3 : Logic  AllPortsSameDT=off  OutDataTypeStr=boolean
  AND5 : Logic  Inputs=3  AllPortsSameDT=off  OutDataTypeStr=boolean
  AND6 : Logic  Inputs=3  AllPortsSameDT=off  OutDataTypeStr=boolean
  Constant : Constant  Value=KDDM_Lv1ErrDetTO_s
  Constant1 : Constant  Value=KDDM_Lv1ErrPassTO_s
  Constant10 : Constant  Value=ENUM_MCUWARN_LV0
  Constant11 : Constant  Value=ENUM_DRIVETRAIN_AWD
  Constant12 : Constant  Value=KDDM_Lv1ErrDTC_cnt
  Constant13 : Constant  Value=ENUM_DRIVETRAIN_AWD
  Constant14 : Constant  Value=ENUM_DRIVETRAIN_FWD
  Constant15 : Constant  Value=ENUM_PWRSTASW_OFF
  Constant18 : Constant  Value=KDDM_Lv1ErrPassTO_s
  Constant2 : Constant  Value=ZERO_INT
  Constant22 : Constant  Value=FALSE
  Constant24 : Constant  Value=TRUE
  Constant25 : Constant  Value=FALSE
  Constant26 : Constant  Value=ENUM_PWRSTASW_OFF
  Constant27 : Constant  Value=FALSE
  Constant3 : Constant  Value=KDDM_FaultLvDiagnosisOffSW_flg
  Constant36 : Constant  Value=ENUM_DCDCFAULTSTA_ANYFAULTLV1
  Constant37 : Constant  Value=ENUM_OBCFAULTSTA_ANYFAULT
  Constant39 : Constant  Value=TRUE
  Constant4 : Constant  Value=ENUM_POWERSTA_OFF
  Constant40 : Constant  Value=KDDM_Lv1ErrDTC_cnt
  Constant5 : Constant  Value=ENUM_SHIFTERERRSTA_PBUTTONFAILURE
  Constant6 : Constant  Value=ENUM_ZONEMALFUNLV_1ST
  Constant7 : Constant  Value=ENUM_ZONEMALFUNLV_1ST
  Constant8 : Constant  Value=ENUM_DRIVETRAIN_RWD
  Constant9 : Constant  Value=ENUM_MCUWARN_LV0
  DTC_Couter : hcu_lib/Basic_Blocks/DTC_Couter
  DTC_Info : hcu_lib/Basic_Blocks/DTC_Info
  Equal : RelationalOperator  Operator=~=  OutDataTypeStr=boolean  RndMeth=Simplest
  Equal{1,4..8,10..12,14..15} (11 alike) : RelationalOperator  Operator===  OutDataTypeStr=boolean  RndMeth=Simplest
  Equal2 : RelationalOperator  Operator=~=  OutDataTypeStr=boolean  RndMeth=Simplest
  Equal3 : RelationalOperator  OutDataTypeStr=boolean  RndMeth=Simplest
  Logical Operator1 : Logic  Inputs=6  AllPortsSameDT=off  OutDataTypeStr=boolean
  Logical Operator16 : Logic  Inputs=6  AllPortsSameDT=off  OutDataTypeStr=boolean
  Logical Operator17 : Logic  Operator=OR  AllPortsSameDT=off  OutDataTypeStr=boolean
  Logical Operator2 : Logic  Operator=OR  AllPortsSameDT=off  OutDataTypeStr=boolean
  Logical Operator6 : Logic  Operator=NOT  AllPortsSameDT=off  OutDataTypeStr=boolean
  Logical Operator8 : Logic  Operator=OR  Inputs=4  AllPortsSameDT=off  OutDataTypeStr=boolean
  NOT{1..3,5..7,9..13,15,17..19,22..24,26,28} (20 alike) : Logic  Operator=NOT  AllPortsSameDT=off  OutDataTypeStr=boolean
  OR : Logic  Operator=OR  Inputs=3  AllPortsSameDT=off  OutDataTypeStr=boolean
  OR1 : Logic  Operator=OR  AllPortsSameDT=off  OutDataTypeStr=boolean
  OR2 : Logic  Operator=OR  Inputs=9  AllPortsSameDT=off  OutDataTypeStr=boolean
  OR3 : Logic  Operator=OR  Inputs=9  AllPortsSameDT=off  OutDataTypeStr=boolean
  Relational Operator : RelationalOperator  Operator=>  OutDataTypeStr=boolean  RndMeth=Simplest
  Relational Operator1 : RelationalOperator  OutDataTypeStr=boolean  RndMeth=Simplest
  Switch{1,4..5,9} (4 alike) : Switch  Criteria=u2 ~= 0
  Terminator : Terminator
  Test Detection Criteria : hcu_lib/Basic_Blocks/Test Detection Criteria
  Timer1 : hcu_lib/Basic_Blocks/Timer
  VDDM_Lv1ErrCFS_flg : Outport
  VDDM_Lv1ErrDTC_raw32 : Outport  Port=2
  wires:
  Switch9/1 -> Test Detection Criteria/1
  Constant22/1 -> Switch9/1
  [VDDM_Lv1ErrCFSRls_flg] -> Switch9/2
  [VDDM_Lv1ErrCFS_flg] -> DTC_Info/3
  [VDDM_Lv1ErrPass_flg] -> DTC_Info/2
  [DTC_clear_request] -> DTC_Info/4
  DTC_Info/1 -> VDDM_Lv1ErrDTC_raw32/1  "VDDM_Lv1ErrDTC_raw32"
  [VDDM_Lv1ErrDet_flg] -> DTC_Info/1
  VDDM_FrVCUNoComCFS_flg/1 -> [VDDM_FrVCUNoComCFS_flg]
  ZoneFrMalfunLevel_enum/1 -> [ZoneFrMalfunLevel_enum]
  VDDM_DrVCUNoComCFS_flg/1 -> [VDDM_DrVCUNoComCFS_flg]
  No_CAN4_BUS_OFF/1 -> [No_CAN4_BUS_OFF]
  VINP_ZoneDrMalfunLevel_enum/1 -> [VINP_ZoneDrMalfunLevel_enum]
  VDDM_Shifter1CSErrCFS_flg/1 -> [VDDM_Shifter1CSErrCFS_flg]
  VDDM_Shifter1RCErrCFS_flg/1 -> [VDDM_Shifter1RCErrCFS_flg]
  VDDM_Shifter1NoComCFS_flg/1 -> [VDDM_Shifter1NoComCFS_flg]
  VINP_ShifterFailsta_enum/1 -> [VINP_ShifterFailsta_enum]
  VDDM_ESC5SigErr_flg/1 -> [VDDM_ESC5SigErr_flg]
  VDDM_ESC1SigErr_flg/1 -> [VDDM_ESC1SigErr_flg]
  No_CAN1_BUS_OFF/1 -> [No_CAN1_BUS_OFF]
  VDDM_C3BMS6CSCFS_flg/1 -> [VDDM_C3BMS6CSCFS_flg]
  VDDM_C3BMS6RCCFS_flg/1 -> [VDDM_C3BMS6RCCFS_flg]
  VDDM_MCUNF1CSErrCFS_flg/1 -> [VDDM_MCUNF1CSErrCFS_flg]
  VDDM_MCUNF1RCErrCFS_flg/1 -> [VDDM_MCUNF1RCErrCFS_flg]
  VDDM_MCUNR1CSErrCFS_flg/1 -> [VDDM_MCUNR1CSErrCFS_flg]
  VDDM_MCUNR1RCErrCFS_flg/1 -> [VDDM_MCUNR1RCErrCFS_flg]
  VDDM_C3CCU2CSCFS_flg/1 -> [VDDM_C3CCU2CSCFS_flg]
  VDDM_C3CCU2RCCFS_flg/1 -> [VDDM_C3CCU2RCCFS_flg]
  Switch1/1 -> Logical Operator6/1, Timer1/2
  Constant15/1 -> Equal2/2
  [VPMM_PwrStaSW_enum] -> Equal2/1
  [VDDM_MCUR1FaultLv1_flg] -> OR3/3
  [VDDM_ESCFaultLv1_flg] -> OR3/6
  Equal2/1 -> Switch1/2
  [VDDM_BMSFaultLv1_flg] -> OR3/5
  [VDDM_MCUF1FaultLv1_flg] -> OR3/4
  [VDDM_DCDCFaultLv1_flg] -> OR3/2
  [VDDM_OBCFaultLv1_flg] -> OR3/1
  OR3/1 -> Switch1/1
  [VDDM_ZoneDrFaultLv1_flg] -> OR3/8
  [VDDM_ShifterFaultLv1_flg] -> OR3/7
  [VDDM_ZoneFrFaultLv1_flg] -> OR3/9
  [VDDM_ZoneFrFaultLv1_flg] -> OR2/9
  [VDDM_ZoneDrFaultLv1_flg] -> OR2/8
  [VDDM_ShifterFaultLv1_flg] -> OR2/7
  [VDDM_ESCFaultLv1_flg] -> OR2/6
  [VDDM_BMSFaultLv1_flg] -> OR2/5
  [VDDM_MCUF1FaultLv1_flg] -> OR2/4
  [VDDM_MCUR1FaultLv1_flg] -> OR2/3
  [VDDM_DCDCFaultLv1_flg] -> OR2/2
  [VDDM_OBCFaultLv1_flg] -> OR2/1
  OR2/1 -> Switch5/1
  [ZoneFrMalfunLevel_enum] -> Equal8/1
  Constant7/1 -> Equal8/2
  Equal8/1 -> AND6/1
  [No_CAN4_BUS_OFF] -> AND6/2
  [VDDM_FrVCUNoComCFS_flg] -> NOT28/1
  NOT28/1 -> AND6/3
  AND6/1 -> [VDDM_ZoneFrFaultLv1_flg]  "VDDM_ZoneFrFaultLv1_flg"
  AND5/1 -> [VDDM_ZoneDrFaultLv1_flg]  "VDDM_ZoneDrFaultLv1_flg"
  NOT26/1 -> AND5/3
  [VDDM_DrVCUNoComCFS_flg] -> NOT26/1
  [No_CAN4_BUS_OFF] -> AND5/2
  Equal1/1 -> AND5/1
  Constant6/1 -> Equal1/2
  [VINP_ZoneDrMalfunLevel_enum] -> Equal1/1
  AND4/1 -> [VDDM_ShifterFaultLv1_flg]  "VDDM_ShifterFaultLv1_flg"
  [VDDM_Shifter1CSErrCFS_flg] -> NOT24/1
  [VDDM_Shifter1RCErrCFS_flg] -> NOT23/1
  [VDDM_Shifter1NoComCFS_flg] -> NOT22/1
  [No_CAN3_BUS_OFF] -> AND4/2
  NOT22/1 -> AND4/3
  NOT23/1 -> AND4/4
  NOT24/1 -> AND4/5
  Relational Operator1/1 -> AND4/1
  Constant5/1 -> Relational Operator1/2
  [VINP_ShifterFailsta_enum] -> Relational Operator1/1
  AND3/1 -> [VDDM_ESCFaultLv1_flg]  "VDDM_ESCFaultLv1_flg"
  OR1/1 -> AND3/2
  [No_CAN1_BUS_OFF] -> AND3/1
  [VDDM_ESC5SigErr_flg] -> OR1/2
  [VDDM_ESC1SigErr_flg] -> OR1/1
  AND2/1 -> [VDDM_BMSFaultLv1_flg]  "VDDM_BMSFaultLv1_flg"
  [VDDM_C3BMS6CSCFS_flg] -> NOT19/1
  [VDDM_C3BMS6RCCFS_flg] -> NOT18/1
  [VDDM_C3BMS6LCCFS_flg] -> NOT17/1
  [No_CAN3_BUS_OFF] -> AND2/2
  NOT17/1 -> AND2/3
  NOT19/1 -> AND2/5
  NOT18/1 -> AND2/4
  OR/1 -> AND2/1
  [VINP_BMSWarn1_flg] -> OR/1
  [VINP_BMSWarn3_flg] -> OR/3
  [VINP_BMSWarn2_flg] -> OR/2
  Equal10/1 -> Logical Operator2/1
  [VINP_MCUWarnFNidec_enum] -> Equal11/1
  Constant14/1 -> Equal10/1
  [VPMM_DrivetrainSelect_enum] -> Equal12/1, Equal10/2
  Constant13/1 -> Equal12/2
  Constant9/1 -> Equal11/2
  Equal11/1 -> Logical Operator1/1
  Equal12/1 -> Logical Operator2/2
  Logical Operator2/1 -> Logical Operator1/6
  NOT13/1 -> Logical Operator1/5
  [No_CAN3_BUS_OFF] -> Logical Operator1/2
  [VDDM_MCUNF1NoComCFS_flg] -> NOT15/1
  NOT15/1 -> Logical Operator1/3
  NOT12/1 -> Logical Operator1/4
  [VDDM_MCUNF1CSErrCFS_flg] -> NOT13/1
  [VDDM_MCUNF1RCErrCFS_flg] -> NOT12/1
  Logical Operator1/1 -> [VDDM_MCUF1FaultLv1_flg]  "VDDM_MCUF1FaultLv1_flg"
  Logical Operator16/1 -> [VDDM_MCUR1FaultLv1_flg]  "VDDM_MCUR1FaultLv1_flg"
  [VDDM_MCUNR1RCErrCFS_flg] -> NOT10/1
  [VDDM_MCUNR1CSErrCFS_flg] -> NOT11/1
  NOT10/1 -> Logical Operator16/4
  NOT9/1 -> Logical Operator16/3
  [VDDM_MCUNR1NoComCFS_flg] -> NOT9/1
  [No_CAN3_BUS_OFF] -> Logical Operator16/2
  NOT11/1 -> Logical Operator16/5
  Logical Operator17/1 -> Logical Operator16/6
  AND1/1 -> [VDDM_DCDCFaultLv1_flg]  "VDDM_DCDCFaultLv1_flg"
  Equal14/1 -> AND1/1
  [No_CAN3_BUS_OFF] -> AND1/2
  NOT7/1 -> AND1/5
  [VDDM_C3CCU2RCCFS_flg] -> NOT6/1
  NOT6/1 -> AND1/4
  [VDDM_C3CCU2LCCFS_flg] -> NOT5/1
  NOT5/1 -> AND1/3
  [VDDM_C3CCU2CSCFS_flg] -> NOT7/1
  AND/1 -> [VDDM_OBCFaultLv1_flg]  "VDDM_OBCFaultLv1_flg"
  NOT3/1 -> AND/5
  NOT2/1 -> AND/4
  NOT1/1 -> AND/3
  [No_CAN3_BUS_OFF] -> AND/2
  [VDDM_C3CCU2LCCFS_flg] -> NOT1/1
  [VDDM_C3CCU2RCCFS_flg] -> NOT2/1
  [VDDM_C3CCU2CSCFS_flg] -> NOT3/1
  Equal15/1 -> AND/1
  [VDDM_Lv1ErrCFS_flg] -> VDDM_Lv1ErrCFS_flg/1
  Constant3/1 -> Logical Operator8/4
  [VDDM_Lv1ErrPass_flg] -> Logical Operator8/3
  Constant2/1 -> Relational Operator/2
  DTC_Couter/1 -> [VDDM_Lv1ErrCFS_flg]  "VDDM_Lv1ErrCFS_flg"
  Switch5/1 -> Switch9/3
  Constant/1 -> Test Detection Criteria/4
  [task_time_s] -> Timer1/3
  No_CAN3_BUS_OFF/1 -> [No_CAN3_BUS_OFF]
  DTC_clear_request/1 -> [DTC_clear_request]
  Equal7/1 -> Logical Operator17/2
  Equal6/1 -> Logical Operator16/1
  Constant10/1 -> Equal6/2
  Constant11/1 -> Equal7/2
  [VPMM_DrivetrainSelect_enum] -> Equal5/2, Equal7/1
  Constant8/1 -> Equal5/1
  [VINP_MCUWarnRNidec_enum] -> Equal6/1
  Equal5/1 -> Logical Operator17/1
  [VPMM_PwrStaSW_enum] -> Equal/1
  [VPMM_PowerSta_enum] -> Equal4/1
  Constant39/1 -> Switch1/3
  Constant37/1 -> Equal15/2
  [VINP_OBCFaultSta_enum] -> Equal15/1
  Constant36/1 -> Equal14/2
  [VINP_DCDCFaultSta_enum] -> Equal14/1
  Constant4/1 -> Equal4/2
  Constant18/1 -> Equal3/2
  Logical Operator6/1 -> Timer1/1
  Constant24/1 -> Switch4/1
  Constant40/1 -> Test Detection Criteria/3
  [task_time_s] -> Test Detection Criteria/2
  Equal/1 -> Switch5/2
  [VDDM_Lv1ErrDet_flg] -> DTC_Couter/1
  Switch4/1 -> [VDDM_Lv1ErrCFSRls_flg]  "VDDM_Lv1ErrCFSRls_flg"
  Constant27/1 -> Switch5/3
  Test Detection Criteria/1 -> [VDDM_Lv1ErrDet_flg]  "VDDM_Lv1ErrDet_flg"
  Constant26/1 -> Equal/2
  [VDDM_Lv1ErrCFSRls_flg] -> DTC_Couter/2
  Logical Operator8/1 -> Switch4/2
  Constant12/1 -> DTC_Couter/3
  Relational Operator/1 -> Terminator/1  "VDDM_Lv1ErrDFS_flg"
  Constant25/1 -> Switch4/3
  Timer1/1 -> Equal3/1
  Equal3/1 -> [VDDM_Lv1ErrPass_flg]  "VDDM_Lv1ErrPass_flg"
  [DTC_clear_request] -> Logical Operator8/2
  DTC_Couter/2 -> Relational Operator/1  "VDDM_Lv1ErrDTC_cnt"
  Constant1/1 -> Timer1/4
  Equal4/1 -> Logical Operator8/1
  VDDM_C3BMS6LCCFS_flg/1 -> [VDDM_C3BMS6LCCFS_flg]
  VINP_OBCFaultSta_enum/1 -> [VINP_OBCFaultSta_enum]
  VINP_MCUWarnFNidec_enum/1 -> [VINP_MCUWarnFNidec_enum]
  VINP_DCDCFaultSta_enum/1 -> [VINP_DCDCFaultSta_enum]
  VINP_BMSWarn3_flg/1 -> [VINP_BMSWarn3_flg]
  VINP_BMSWarn2_flg/1 -> [VINP_BMSWarn2_flg]
  VINP_BMSWarn1_flg/1 -> [VINP_BMSWarn1_flg]
  VDDM_MCUNF1NoComCFS_flg/1 -> [VDDM_MCUNF1NoComCFS_flg]
  VDDM_MCUNR1NoComCFS_flg/1 -> [VDDM_MCUNR1NoComCFS_flg]
  VINP_MCUWarnRNidec_enum/1 -> [VINP_MCUWarnRNidec_enum]
  VPMM_DrivetrainSelect_enum/1 -> [VPMM_DrivetrainSelect_enum]
  VDDM_C3CCU2LCCFS_flg/1 -> [VDDM_C3CCU2LCCFS_flg]
  VPMM_PowerSta_enum/1 -> [VPMM_PowerSta_enum]
  VPMM_PwrStaSW_enum/1 -> [VPMM_PwrStaSW_enum]
  task_time_s/1 -> [task_time_s]
